simulink model "system2"  (Simulink 4.00)
settings: Solver=ode45  StartTime=0.0  StopTime=10.0  RelTol=1e-3
libraries: cstblocks x3, simulink_extras x1
settings Model: LastModifiedBy=Administrator  BlockReductionOpt=off

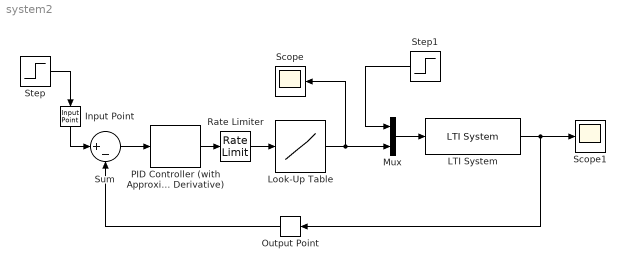
== system system2 ==
  Input Point : cstblocks/Input Point  Orientation=down
  LTI System : cstblocks/LTI System  sys=my_sys1  IC=0
  Look-Up Table : Lookup  InputValues=[-50. -15,- 10, 0, 10, 15, 50]  OutputValues=[-15, -12, -10, 0, 10, 12, 15]
  Mux : Mux  Inputs=2
  Output Point : cstblocks/Output Point  Orientation=left
  PID Controller (with Approximate Derivative) : simulink_extras/Additional Linear/PID Controller (with Approximate Derivative)  P=10  I=8  D=1  N=20
  Rate Limiter : RateLimiter  RisingSlewLimit=50  FallingSlewLimit=-50
  Scope : Scope
      settings: TimeRange=auto  YMin=-5  YMax=5  SaveToWorkspace=off  SaveName=ScopeData  LimitDataPoints=on  MaxDataPoints=5000
  Scope1 : Scope
      settings: TimeRange=auto  YMin=-5  YMax=5  SaveToWorkspace=off  LimitDataPoints=on  MaxDataPoints=5000
  Step : Step  Time=0  Before=0  After=1  SampleTime=0
  Step1 : Step  Orientation=left  Time=0  Before=0  After=0  SampleTime=0
  Sum : Sum  Inputs=|+-  SaturateOnIntegerOverflow=on
  wires:
  Step/1 -> Input Point/1
  Sum/1 -> PID Controller (with Approximate Derivative)/1
  PID Controller (with Approximate Derivative)/1 -> Rate Limiter/1
  Rate Limiter/1 -> Look-Up Table/1
  Input Point/1 -> Sum/1
  Output Point/1 -> Sum/2
  Look-Up Table/1 -> Scope/1, Mux/2
  Mux/1 -> LTI System/1
  Step1/1 -> Mux/1
  LTI System/1 -> Output Point/1, Scope1/1
